simulink model "DoubleCheck_simulink"  (R2018b)
settings: Solver=ode45  StartTime=0.0  StopTime=10  RelTol=1e-4
values from neighbouring files (symbols this model uses):
  fs = 100    [DoubleCheck.m]    (also in ExcitationSignal.m; MainRoute.m)
libraries: cstblocks x4
settings Model: Creator=mahao  LastModifiedBy=mahao

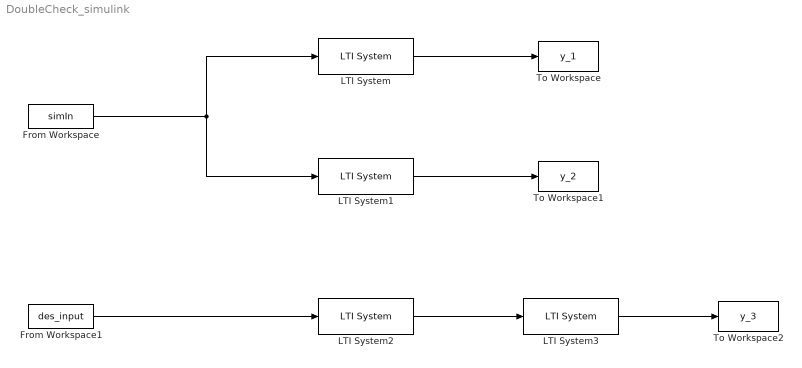
== system DoubleCheck_simulink ==
  From Workspace : FromWorkspace  VariableName=simIn  SampleTime=1/fs
  From Workspace1 : FromWorkspace  VariableName=des_input  SampleTime=1/fs
  LTI System : cstblocks/LTI System  sys=G  IC=[]
  LTI System1 : cstblocks/LTI System  sys=G_delay  IC=[]
  LTI System2 : cstblocks/LTI System  sys=G_inv  IC=[]
  LTI System3 : cstblocks/LTI System  sys=G_delay  IC=[]
  To Workspace : ToWorkspace  VariableName=y_1  SampleTime=1/fs
  To Workspace1 : ToWorkspace  VariableName=y_2  SampleTime=1/fs
  To Workspace2 : ToWorkspace  VariableName=y_3  SampleTime=1/fs
  wires:
  LTI System/1 -> To Workspace/1
  LTI System1/1 -> To Workspace1/1
  From Workspace/1 -> LTI System/1, LTI System1/1
  From Workspace1/1 -> LTI System2/1
  LTI System2/1 -> LTI System3/1
  LTI System3/1 -> To Workspace2/1
